simulink model "controle_arx"  (R2017a)
settings: Solver=VariableStepAuto  StartTime=0.0  StopTime=10  RelTol=1e-3
values from neighbouring files (symbols this model uses):
  A1 = [1.49897851716768 -0.658867228285944 0.452612718877348 -0.341574690861248 -0.155335749359606 0.126936388999114;1 0 0 0 0 0;0 1 0 0 0 0;0 0 1 0 0 0;0 0 0 1 0 0;0 0 0 0 1 0]    [controle_arx2.m]    (also in controle_arx3.m = [1.55060903848634 -0.760133957710275 0.532127876964906 -0.48; controle_arx4.m = [1.55060903848634 -0.760133957710275 0.532127876964906 -0.48; controle_arxsim.m = [1.01084017733551 -0.453091619596496 0.434089118323531;1 0 0)
  B1 = [1;0;0;0;0;0]    [controle_arx2.m]    (also in controle_arx3.m = [1;0;0;0;0]; controle_arx4.m = [1;0;0;0;0]; controle_arxsim.m = [1;0;0])
  C1 = [-0.00935904114014577 0.0183508990918752 0.00773761149536270 0.0402641014305046 0.0383901175590003 -0.000489474738462096]    [controle_arx2.m]    (also in controle_arx3.m = [-0.00854754496452607 0.0165466900077137 0.00409300990441686; controle_arx4.m = [-0.00854754496452607 0.0165466900077137 0.00409300990441686; controle_arxsim.m = [-0.00201156891470309 0.00830655499096105 -0.001591481446917)
  D1 = [-0.00385606320080141]    [controle_arx2.m]    (also in controle_arx3.m = [-0.00293485774062023]; controle_arx4.m = [-0.00293485774062023]; controle_arxsim.m = [-0.00366625510693185])
  k1 = kb*inv(t1)    [controle_arx2.m]    (also in controle_arx3.m; controle_arx4.m; controle_arxsim.m)
  l1 = inv(t2)*lb    [controle_arx2.m]    (also in controle_arx3.m; controle_arx4.m)
settings Model: Creator=Vicente  LastModifiedBy=Vicente

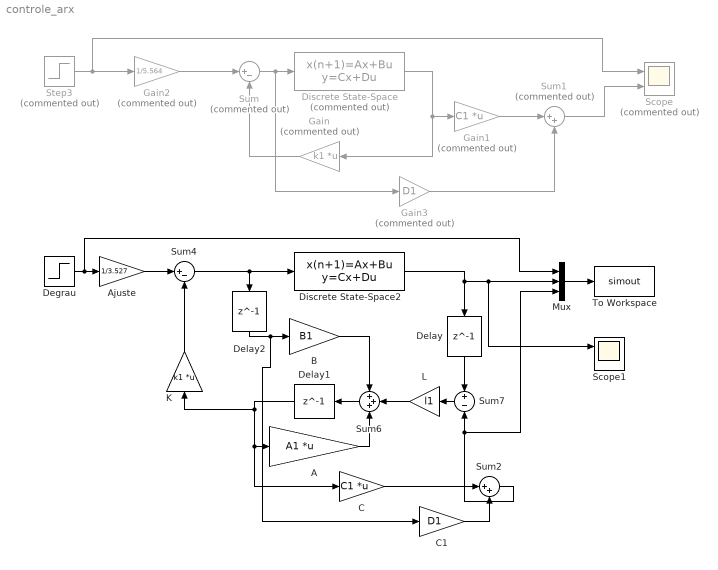
== system controle_arx ==
  A : Gain  Gain=A1  Multiplication=Matrix(K*u)
  Ajuste : Gain  Gain=1/3.527
  B : Gain  Gain=B1
  C : Gain  Gain=C1  Multiplication=Matrix(K*u)
  C1 : Gain  Gain=D1
  Degrau : Step  Time=4  Before=1  After=0.8  SampleTime=0
  Delay : Delay  DelayLength=1  InitialCondition=0
  Delay1 : Delay  DelayLength=1  InitialCondition=0
  Delay2 : Delay  DelayLength=1  InitialCondition=0
  Discrete State-Space : DiscreteStateSpace  Commented=on  A=A1  B=B1  C=eye(5)  D=[0;0;0;0;0]  SampleTime=0.05
  Discrete State-Space2 : DiscreteStateSpace  A=A1  B=B1  C=C1  D=D1  SampleTime=0.05
  Gain : Gain  Commented=on  Gain=k1  Multiplication=Matrix(K*u)
  Gain1 : Gain  Commented=on  Gain=C1  Multiplication=Matrix(K*u)
  Gain2 : Gain  Commented=on  Gain=1/5.564
  Gain3 : Gain  Commented=on  Gain=D1
  K : Gain  Gain=k1  Multiplication=Matrix(K*u)
  L : Gain  Gain=l1
  Mux : Mux  Inputs=3
  Scope : Scope  Commented=on  NumInputPorts=2
  Scope1 : Scope  NumInputPorts=2
  Step3 : Step  Commented=on  Time=0  SampleTime=0
  Sum : Sum  Commented=on  Inputs=|+-
  Sum1 : Sum  Commented=on  Inputs=|++
  Sum2 : Sum  Inputs=|++
  Sum4 : Sum  Inputs=|+-
  Sum6 : Sum  Inputs=+++
  Sum7 : Sum  Inputs=+|-
  To Workspace : ToWorkspace  VariableName=simout  SaveFormat=Timeseries  SampleTime=0.05
  wires:
  Discrete State-Space/1 -> Gain1/1, Gain/1
  Sum/1 -> Gain3/1, Discrete State-Space/1
  Gain1/1 -> Sum1/1
  Gain/1 -> Sum/2
  Step3/1 -> Gain2/1, Scope/1
  Discrete State-Space2/1 -> Scope1/1, Mux/2, Delay/1
  Degrau/1 -> Mux/1, Ajuste/1
  Delay/1 -> Sum7/1
  L/1 -> Sum6/2
  Sum6/1 -> Delay1/1
  A/1 -> Sum6/3
  Delay2/1 -> C1/1, B/1
  B/1 -> Sum6/1
  Delay1/1 -> K/1, A/1, C/1
  C/1 -> Sum2/1
  Sum1/1 -> Scope/2
  Gain3/1 -> Sum1/2
  Sum7/1 -> L/1
  K/1 -> Sum4/2
  Gain2/1 -> Sum/1
  Ajuste/1 -> Sum4/1
  Sum4/1 -> Delay2/1, Discrete State-Space2/1
  C1/1 -> Sum2/2
  Sum2/1 -> Mux/3, Sum7/2
  Mux/1 -> To Workspace/1
